simulink model "anguloRecto1_1"  (R2014a)
settings: Solver=ode45  StartTime=0.0  StopTime=10.0  RelTol=1e-3
undefined symbols (not defined in the file): sigbuilder_block
libraries: simulink x1
settings Model: Creator=PedroBarquin  LastModifiedBy=PedroBarquin

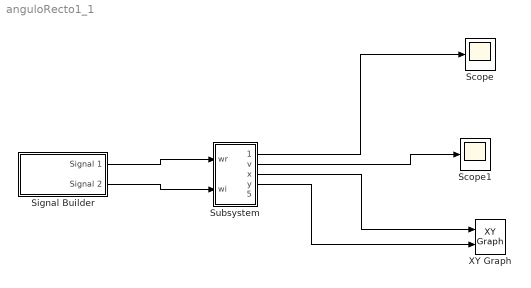
== system anguloRecto1_1 ==
  Scope : Scope
  Scope1 : Scope
  Signal Builder : Subsystem  Tag=STV Subsys  LoadFcn=sigbuilder_block('load');  StartFcn=sigbuilder_block('start');  StopFcn=sigbuilder_block('stop');  ClipboardFcn=sigbuilder_block('clipboard');  mask(Sigbuilder block){}
      mask help: Simulink:masks:SigbuilderBlock_MD
      mask init:
      | if ~strcmp(get_param(bdroot(gcbh),'SimulationStatus'),'stopped') tuvar = sigbuilder_block('maskInit'); end
      settings: CopyFcn=sigbuilder_block('copy');  DeleteFcn=sigbuilder_block('delete');  ModelCloseFcn=sigbuilder_block('modelClose');  PreSaveFcn=sigbuilder_block('preSave');  PauseFcn=sigbuilder_block('pause');  ContinueFcn=sigbuilder_block('continue');  NameChangeFcn=sigbuilder_block('namechange');  OpenFcn=sigbuilder_block('open',[21.75 40.5 496.5 435 ]);  CloseFcn=sigbuilder_block('close');
      mask Display: plot(0, 0, 100, 100,[2, 2, 32, 32, 2], [68, 8, 8, 68, 68],[32, 2], [38, 38], [32, 19, 2],[53, 60, 44], [32, 17, 17, 2],[16, 16, 31, 31]);txt = getActiveGroup(gcbh);text(2, 100, txt,'verticalAlignment', 'top');
  Subsystem : Subsystem  mask{r=1, L=1, x_0=0, y_0=0, theta_0=0}
  XY Graph : simulink/Sinks/XY Graph  xmin=-2  xmax=2  ymin=-2  ymax=2  st=-1
  wires:
  Subsystem/1("omega ") -> Scope/1
  Subsystem/2("v ") -> Scope1/1
  Subsystem/3("x ") -> XY Graph/1
  Subsystem/4("y ") -> XY Graph/2
  Signal Builder/1(Signal 1) -> Subsystem/1("wr ")
  Signal Builder/2(Signal 2) -> Subsystem/2(wi)

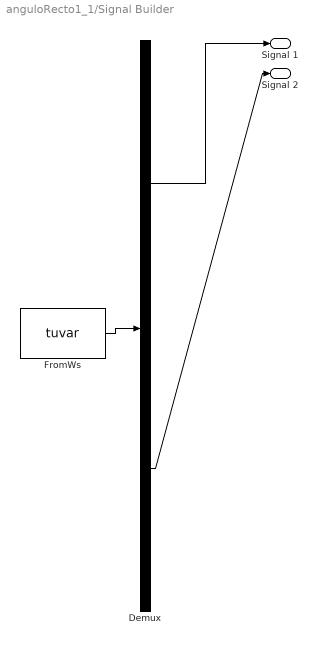
== system anguloRecto1_1/Signal Builder ==
  Demux : Demux  Tag=STV Demux  Outputs=2
  FromWs : FromWorkspace  Tag=STV FromWs  VariableName=tuvar  SampleTime=0
      SigBuilderData=|
      | common.afterFinalStr = 'Extrapolate'
      | common.sampleTime = 0
      | dataSet.timeRange = [0 10]
      | dataSet.name = 'Group 1'
      | sbobj.Groups.Name = 'Group 1'
      | sbobj.Groups.Signals(1).Name = 'Signal 1'
      | sbobj.Groups.Signals(1).XData = [0 0.5 0.5 1.5 10]
      | sbobj.Groups.Signals(1).YData = [0 0 1 1 1]
      | sbobj.Groups.Signals(2).Name = 'Signal 2'
      | sbobj.Groups.Signals(2).XData = [0 0.5 0.5 1 1 1.785 1.785 10]
      | sbobj.Groups.Signals(2).YData = [0 0 1 1 -1 -1 1 1]
  Signal 1 : Outport  Tag=STV Outport
  Signal 2 : Outport  Tag=STV Outport  Port=2
  wires:
  Demux/1 -> Signal 1/1
  FromWs/1 -> Demux/1
  Demux/2 -> Signal 2/1

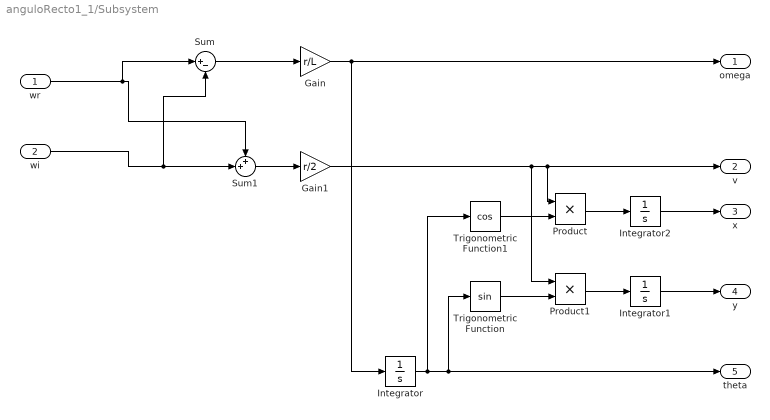
== system anguloRecto1_1/Subsystem ==
  "wr " : Inport
  wi : Inport  Port=2
  Gain : Gain  Gain=r/L
  Gain1 : Gain  Gain=r/2
  Integrator : Integrator  InitialCondition=theta_0
  Integrator1 : Integrator  InitialCondition=y_0
  Integrator2 : Integrator  InitialCondition=x_0
  Product : Product
  Product1 : Product
  Sum : Sum  Inputs=|+-
  Sum1 : Sum  Inputs=++|
  Trigonometric Function : Trigonometry
  Trigonometric Function1 : Trigonometry  Operator=cos
  "omega " : Outport
  "v " : Outport  Port=2
  "x " : Outport  Port=3
  "y " : Outport  Port=4
  "theta " : Outport  Port=5
  wires:
  Gain/1 -> "omega "/1, Integrator/1
  Sum/1 -> Gain/1
  Gain1/1 -> Product1/1, "v "/1, Product/1
  Sum1/1 -> Gain1/1
  wi/1 -> Sum/2, Sum1/2
  "wr "/1 -> Sum/1, Sum1/1
  Trigonometric Function/1 -> Product1/2
  Trigonometric Function1/1 -> Product/2
  Product1/1 -> Integrator1/1
  Integrator/1 -> Trigonometric Function1/1, "theta "/1, Trigonometric Function/1
  Integrator1/1 -> "y "/1
  Product/1 -> Integrator2/1
  Integrator2/1 -> "x "/1
